simulink model "controllability_test_simulation"  (R2021a)
settings: Solver=VariableStepAuto  StartTime=0.0  StopTime=25  RelTol=1e-3
values from neighbouring files (symbols this model uses):
  A = [0 1 0 0 ... (first row only)    [Controllability_of_a_Linear_System.m]    (also in Full_State_Feedback_Control_Design.m = [0 3;2 4]; Implementation_Issues_with_a_FSFB.m = [0 1 0; Introduction_to_Full_State_Feedback_COntrol.m = [0 3;2 4]; Introduction_to_LQR_control.m = [0 1)
  B = [0 ... (first row only)    [Controllability_of_a_Linear_System.m]    (also in Full_State_Feedback_Control_Design.m = [-2 1; 1 1]; Implementation_Issues_with_a_FSFB.m = [0 0; Introduction_to_Full_State_Feedback_COntrol.m = [-2 1; 1 1]; Introduction_to_LQR_control.m)
settings Model: Creator=subhi  LastModifiedBy=subhi

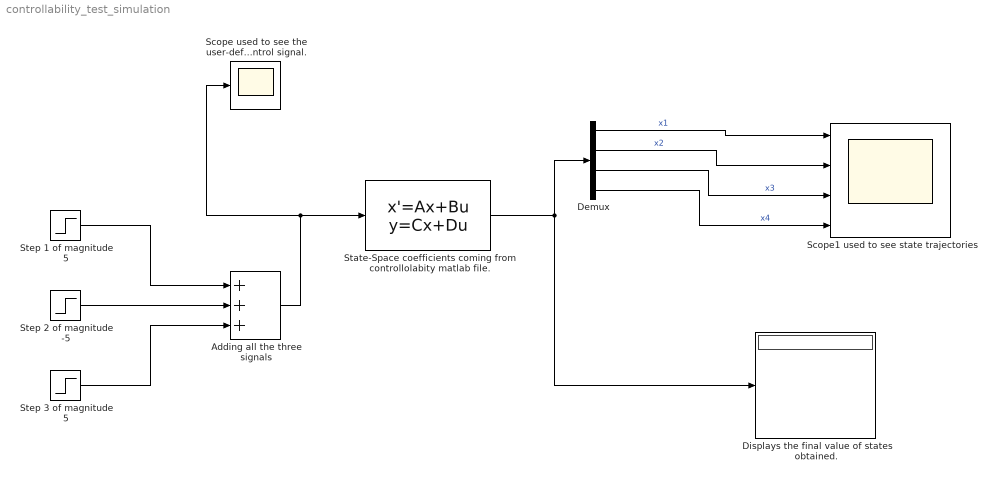
== system controllability_test_simulation ==
  Adding all the three signals : Sum  Inputs=+++
  Demux : Demux
  Displays the final value of states obtained. : Display
  Scope used to see the user-defined control signal. : Scope
  Scope1 used to see state trajectories : Scope  NumInputPorts=4
  State-Space coefficients coming from controllolabity matlab file. : StateSpace  A=A  B=B  C=eye(4)  D=zeros(4,1)  InitialCondition=zeros(4,1)
  "Step 1 of magnitude 5 " : Step  Time=5  After=5  SampleTime=1
  Step 2 of magnitude -5 : Step  Time=8  After=-5  SampleTime=0
  Step 3 of magnitude 5 : Step  Time=14  After=5  SampleTime=0
  wires:
  State-Space coefficients coming from controllolabity matlab file./1 -> Displays the final value of states obtained./1, Demux/1
  Demux/1 -> Scope1 used to see state trajectories/1  "x1"
  Demux/4 -> Scope1 used to see state trajectories/4  "x4"
  Demux/3 -> Scope1 used to see state trajectories/3  "x3"
  Demux/2 -> Scope1 used to see state trajectories/2  "x2"
  "Step 1 of magnitude 5 "/1 -> Adding all the three signals/1
  Step 2 of magnitude -5/1 -> Adding all the three signals/2
  Step 3 of magnitude 5/1 -> Adding all the three signals/3
  Adding all the three signals/1 -> Scope used to see the user-defined control signal./1, State-Space coefficients coming from controllolabity matlab file./1
